simulink model "DCmachineChange0"  (R2017b)
settings: Solver=VariableStepAuto  StartTime=0.0  StopTime=10.0  MaxStep=1e-4  RelTol=1e-3
libraries: powerlib x12, powerlib_extras x1
settings Model: Creator=80573  LastModifiedBy=80573

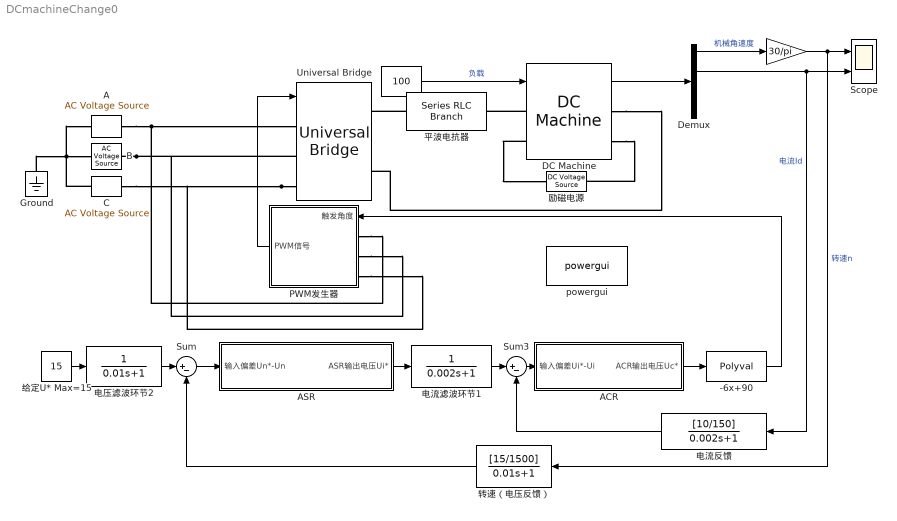
== system DCmachineChange0 ==
  " " : Gain  Gain=30/pi  SaturateOnIntegerOverflow=on  OutDataTypeStr=Inherit: Same as input  ParamDataTypeStr=Inherit: Same as input
  " " : Constant  Value=100
  -6x+90 : Polyval  Coefs=[-6 90]
  A : powerlib/Electrical Sources/AC Voltage Source  Amplitude=220  Phase=0  Frequency=50  SampleTime=0  Measurements=None  BusType=swing  Pref=10e3  Qref=0  Qmin=-inf  Qmax=+inf
  ACR : Subsystem
  ASR : Subsystem
  B : powerlib/Electrical Sources/AC Voltage Source  Amplitude=220  Phase=240  Frequency=50  SampleTime=0  Measurements=None  BusType=swing  Pref=10e3  Qref=0  Qmin=-inf  Qmax=+inf
  C : powerlib/Electrical Sources/AC Voltage Source  Amplitude=220  Phase=120  Frequency=50  SampleTime=0  Measurements=None  BusType=swing  Pref=10e3  Qref=0  Qmin=-inf  Qmax=+inf
  DC Machine : powerlib/Machines/DC Machine  PresetModel=No  MechanicalLoad=Torque TL  FieldType=Wound  ShowDetailedParameters=on  MeasurementBus=off  RLa="[0.16  0.0028]"  RLf=[56.25 0]  Laf=0.404  MachineConstant=Torque constant (N.m/A)  Ke=1.8  Kt=1.8  J=0.671  Bm=0  Tf=0  w0=0  Ifinit=1  TsPowergui=0  TsBlock=-1
  Demux : Demux
  Ground : powerlib/Elements/Ground  LConnTagsString=a
  PWM发生器 : Subsystem
  Scope : Scope  NumInputPorts=2
  Sum : Sum  Inputs=|+-
  Sum3 : Sum  Inputs=|+-
  Universal Bridge : powerlib/Power Electronics/Universal Bridge  Arms=3  SnubberResistance=1e5  SnubberCapacitance=inf  Device=Thyristors  Ron=0.5  Lon=0  ForwardVoltages="[  0  0  ]"  ForwardVoltage=0  GTOparameters=[ 10e-6 , 20e-6 ]  IGBTparameters=[ 1e-6 , 2e-6 ]  Measurements=None  Measurements_2=None  converterType=Rectifier
  powergui : powerlib/powergui  Priority=1  SimulationMode=Continuous  SampleTime=50e-6  frequency=60  Iterations=50  frequencyindice=0  Pbase=100e6  ErrMax=1e-4  UnitsV=kV  UnitsW=MW  buscounter=0  FunctionMessages=off  echomessages=off  EnableUseOfTLC=off  CurrentSourceSwitches=off  DisableSnubberDevices=off  DisableRonSwitches=off  DisableVfSwitches=off  DisplayEquations=off  SolverType=Tustin/Backward Euler (TBE)  Interpol=off  ExternalGateDelay=off  methode=off  Ts=100  x0status=blocks  SPID=on  SwTol=0  HookPort=off  RestoreLinks=warning  ResistiveCurrentMeasurement=off  Frange=[0:2:500]  Ylog=off  Xlog=on  ShowGrid=off  save=off  variable=ZData  structure=0  ZoomFFT=off  StartTime=0.0  cycles=1  DisplayStyle=1  fundamental=60  FreqAxis=off  MaxFrequency=1000  frequencyindicesteady=1  RmsSteady=1  display=off
  励磁电源 : powerlib/Electrical Sources/DC Voltage Source  Amplitude=180  Measurements=None
  平波电抗器 : powerlib/Elements/Series RLC Branch  LConnTagsString=__new0  RConnTagsString=__new0  BranchType=L  Resistance=0.001  Inductance=20e-3  SetiL0=off  InitialCurrent=0  Capacitance=1e-6  Setx0=off  InitialVoltage=0  Measurements=None
  电压滤波环节2 : TransferFcn  Denominator=[0.01 1]
  电流反馈 : TransferFcn  Numerator=[10/150]  Denominator=[0.002 1]
  电流滤波环节1 : TransferFcn  Denominator=[0.002 1]
  给定U* Max=15 : Constant  Value=15
  转速（电压反馈） : TransferFcn  Numerator=[15/1500]  Denominator=[0.01 1]
  wires:
  DC Machine/1 -> Demux/1
  ACR/1(ACR输出电压Uc*) -> -6x+90/1
  Sum3/1 -> ACR/1(输入偏差Ui*-Ui)
  给定U* Max=15/1 -> 电压滤波环节2/1
  ASR/1(ASR输出电压Ui*) -> 电流滤波环节1/1
  -6x+90/1 -> PWM发生器/1(触发角度)
  Sum/1 -> ASR/1(输入偏差Un*-Un)
  " "/1 -> Scope/1, 转速（电压反馈）/1  "转速n"
  电流滤波环节1/1 -> Sum3/1
  电流反馈/1 -> Sum3/2
  转速（电压反馈）/1 -> Sum/2
  Demux/1 -> " "/1  "机械角速度"
  " "/1 -> DC Machine/1  "负载"
  PWM发生器/1(PWM信号) -> Universal Bridge/1
  电压滤波环节2/1 -> Sum/1
  Demux/2 -> Scope/2, 电流反馈/1  "电流Id"
  connections:
  B/RConn1 -- Universal Bridge/LConn2 -- PWM发生器/LConn2
  Universal Bridge/LConn3 -- C/RConn1 -- PWM发生器/LConn3
  PWM发生器/LConn1 -- A/RConn1 -- Universal Bridge/LConn1
  Ground/LConn1 -- A/LConn1 -- C/LConn1 -- B/LConn1
  DC Machine/RConn1 -- Universal Bridge/RConn2
  平波电抗器/LConn1 -- Universal Bridge/RConn1
  DC Machine/LConn2 -- 励磁电源/RConn1
  DC Machine/LConn1 -- 平波电抗器/RConn1
  DC Machine/RConn2 -- 励磁电源/LConn1

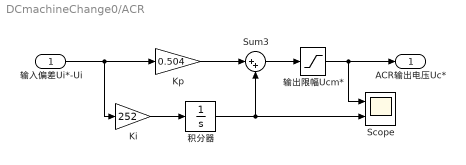
== system DCmachineChange0/ACR ==
  输入偏差Ui*-Ui : Inport
  Ki : Gain  Gain=252
  Kp : Gain  Gain=0.504
  Scope : Scope  NumInputPorts=2
  Sum3 : Sum  Inputs=|++
  积分器 : Integrator  LimitOutput=on  UpperSaturationLimit=12  LowerSaturationLimit=-12
  输出限幅Ucm* : Saturate  UpperLimit=10  LowerLimit=-10
  ACR输出电压Uc* : Outport
  wires:
  积分器/1 -> Sum3/2, Scope/2
  Ki/1 -> 积分器/1
  Kp/1 -> Sum3/1
  输入偏差Ui*-Ui/1 -> Ki/1, Kp/1
  Sum3/1 -> 输出限幅Ucm*/1
  输出限幅Ucm*/1 -> Scope/1, ACR输出电压Uc*/1

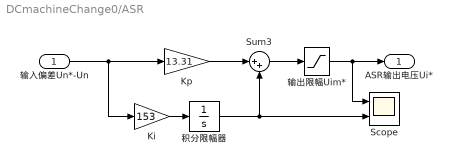
== system DCmachineChange0/ASR ==
  输入偏差Un*-Un : Inport
  Ki : Gain  Gain=153
  Kp : Gain  Gain=13.31
  Scope : Scope  NumInputPorts=2
  Sum3 : Sum  Inputs=|++
  积分限幅器 : Integrator  LimitOutput=on  UpperSaturationLimit=9  LowerSaturationLimit=-9
  输出限幅Uim* : Saturate  UpperLimit=8  LowerLimit=-8
  ASR输出电压Ui* : Outport
  wires:
  积分限幅器/1 -> Scope/2, Sum3/2
  Ki/1 -> 积分限幅器/1
  Kp/1 -> Sum3/1
  输入偏差Un*-Un/1 -> Ki/1, Kp/1
  Sum3/1 -> 输出限幅Uim*/1
  输出限幅Uim*/1 -> Scope/1, ASR输出电压Ui*/1

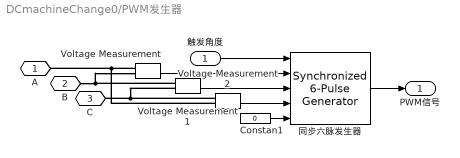
== system DCmachineChange0/PWM发生器 ==
  触发角度 : Inport
  Constan1 : Constant  Value=0
  Voltage Measurement : powerlib/Measurements/Voltage Measurement  PhasorSimulation=off  OutputType=Complex  PSBequivalent=0
  Voltage Measurement1 : powerlib/Measurements/Voltage Measurement  PhasorSimulation=off  OutputType=Complex  PSBequivalent=0
  Voltage Measurement2 : powerlib/Measurements/Voltage Measurement  PhasorSimulation=off  OutputType=Complex  PSBequivalent=0
  同步六脉发生器 : powerlib_extras/Control  Blocks/Synchronized 6-Pulse Generator  freq=50  pwidth=10  Double_Pulse=on
  A : PMIOPort  Port=1  Side=Left
  B : PMIOPort  Port=2  Side=Left
  C : PMIOPort  Port=3  Side=Left
  PWM信号 : Outport
  wires:
  同步六脉发生器/1 -> PWM信号/1
  Voltage Measurement/1 -> 同步六脉发生器/2
  Voltage Measurement1/1 -> 同步六脉发生器/3
  Voltage Measurement2/1 -> 同步六脉发生器/4
  触发角度/1 -> 同步六脉发生器/1
  Constan1/1 -> 同步六脉发生器/5
  connections:
  Voltage Measurement/LConn1 -- Voltage Measurement2/LConn2 -- A/RConn1
  B/RConn1 -- Voltage Measurement/LConn2 -- Voltage Measurement1/LConn1
  Voltage Measurement1/LConn2 -- Voltage Measurement2/LConn1 -- C/RConn1
